simulink model "Funtivities_pt2"  (R2023b)
settings: Solver=VariableStepAuto  StartTime=0.0  StopTime=2  RelTol=1e-3
model workspace: external: MATLAB File D:\College\Senior 2\GP\Delta\Design\INSHALLAAHHHHH\SSCPE\Funtivities_pt2_DataFile.m (data not in the file)
undefined symbols (not defined in the file or in its folder): smiData, X, Y, Z
libraries: sm_lib x234, nesl_utility x7, simulink_extras x6
(part 1 of 6)
settings Model: Creator=Dell  LastModifiedBy=Dell

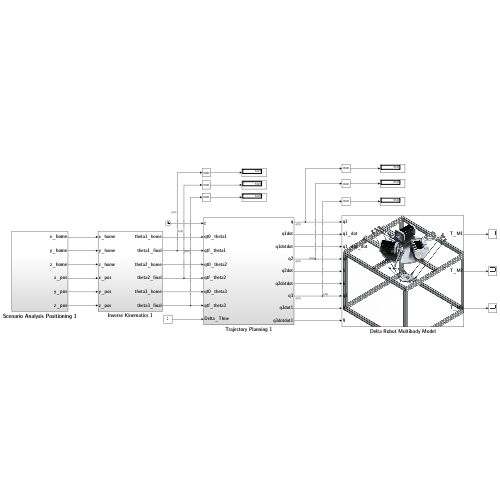
[thumbnail: Simulink's stored preview of the top-level diagram]
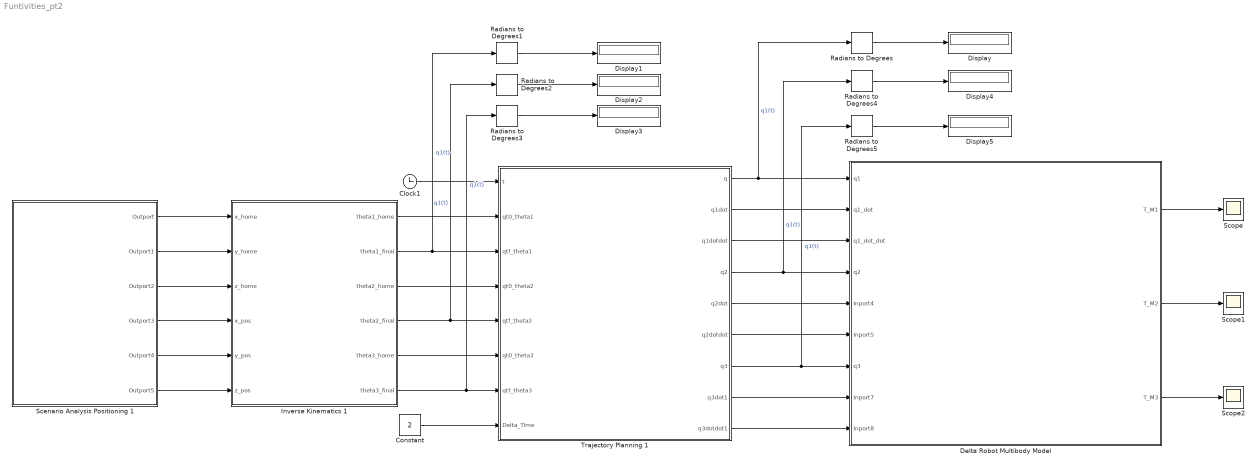
== system Funtivities_pt2 ==
  Clock1 : Clock
      settings: Decimation=5
  Constant : Constant  Value=2
  Delta Robot Multibody Model : Subsystem
      mask Display: image('r10.png');
  Display{,1..5} (6 alike) : Display
  Inverse Kinematics 1 : Subsystem
  Radians to Degrees{,1..5} (6 alike) : simulink_extras/Transformations/Radians to Degrees
  Scenario Analysis Positioning 1 : Subsystem
  Scope : Scope
  Scope1 : Scope
  Scope2 : Scope
  Trajectory Planning 1 : Subsystem
  wires:
  Radians to Degrees/1 -> Display/1
  Radians to Degrees1/1 -> Display1/1
  Trajectory Planning 1/8(q3dot1) -> Delta Robot Multibody Model/8(Inport7)
  Trajectory Planning 1/5(q2dot) -> Delta Robot Multibody Model/5(Inport4)
  Trajectory Planning 1/9(q3dotdot1) -> Delta Robot Multibody Model/9(Inport8)
  Trajectory Planning 1/6(q2dotdot) -> Delta Robot Multibody Model/6(Inport5)
  Trajectory Planning 1/1(q) -> Delta Robot Multibody Model/1(q1), Radians to Degrees/1  "q1(t)"
  Trajectory Planning 1/2(q1dot) -> Delta Robot Multibody Model/2(q1_dot)
  Scenario Analysis Positioning 1/1(Outport) -> Inverse Kinematics 1/1(x_home)
  Inverse Kinematics 1/3(theta2_home) -> Trajectory Planning 1/4(qt0_theta2)
  Scenario Analysis Positioning 1/4(Outport3) -> Inverse Kinematics 1/4(x_pos)
  Inverse Kinematics 1/5(theta3_home) -> Trajectory Planning 1/6(qt0_theta3)
  Trajectory Planning 1/3(q1dotdot) -> Delta Robot Multibody Model/3(q1_dot_dot)
  Scenario Analysis Positioning 1/6(Outport5) -> Inverse Kinematics 1/6(z_pos)
  Inverse Kinematics 1/1(theta1_home) -> Trajectory Planning 1/2(qt0_theta1)
  Scenario Analysis Positioning 1/2(Outport1) -> Inverse Kinematics 1/2(y_home)
  Scenario Analysis Positioning 1/3(Outport2) -> Inverse Kinematics 1/3(z_home)
  Scenario Analysis Positioning 1/5(Outport4) -> Inverse Kinematics 1/5(y_pos)
  Clock1/1 -> Trajectory Planning 1/1(t)
  Constant/1 -> Trajectory Planning 1/8(Delta_TIme)
  Inverse Kinematics 1/2(theta1_final) -> Radians to Degrees1/1, Trajectory Planning 1/3(qtf_theta1)  "q1(t)"
  Inverse Kinematics 1/4(theta2_final) -> Radians to Degrees2/1, Trajectory Planning 1/5(qtf_theta2)  "q1(t)"
  Radians to Degrees2/1 -> Display2/1
  Inverse Kinematics 1/6(theta3_final) -> Radians to Degrees3/1, Trajectory Planning 1/7(qtf_theta3)  "q1(t)"
  Radians to Degrees3/1 -> Display3/1
  Radians to Degrees4/1 -> Display4/1
  Trajectory Planning 1/4(q2) -> Radians to Degrees4/1, Delta Robot Multibody Model/4(q2)  "q1(t)"
  Trajectory Planning 1/7(q3) -> Radians to Degrees5/1, Delta Robot Multibody Model/7(q3)  "q1(t)"
  Radians to Degrees5/1 -> Display5/1
  Delta Robot Multibody Model/1(T_M1) -> Scope/1
  Delta Robot Multibody Model/2(T_M2) -> Scope1/1
  Delta Robot Multibody Model/3(T_M3) -> Scope2/1
